simulink model "ES008A_PwrSply"  (R2013b)
settings: Solver=FixedStepDiscrete  SolverMode=SingleTasking  StartTime=0.0  StopTime=1  FixedStep=0.002  RelTol=1e-3
values from neighbouring files (symbols this model uses):
  DiagcReg0Err = DataDict.NTC    [ES008A_PwrSply_DataDict.m]
  DiagcReg1Err = DataDict.NTC    [ES008A_PwrSply_DataDict.m]
  PWRSPLYDIAGREG0READVAL_CNT_U16 = DataDict.Constant    [ES008A_PwrSply_DataDict.m]
  PWRSPLYDIAGREG1READVAL_CNT_U16 = DataDict.Constant    [ES008A_PwrSply_DataDict.m]
  PwrSplyNtc0x07BFailStep = DataDict.Calibration    [ES008A_PwrSply_DataDict.m]
  PwrSplyNtc0x07BPassStep = DataDict.Calibration    [ES008A_PwrSply_DataDict.m]
  PwrSplyNtc0x07CFailStep = DataDict.Calibration    [ES008A_PwrSply_DataDict.m]
  PwrSplyNtc0x07CPassStep = DataDict.Calibration    [ES008A_PwrSply_DataDict.m]
  PwrSplyNtc0x07DFailStep = DataDict.Calibration    [ES008A_PwrSply_DataDict.m]
  PwrSplyNtc0x07DPassStep = DataDict.Calibration    [ES008A_PwrSply_DataDict.m]
  PWRSPLYOUTPENAWRVAL_CNT_U16 = DataDict.Constant    [ES008A_PwrSply_DataDict.m]
  PWRSPLYVRFYRESREG0READVAL_CNT_U16 = DataDict.Constant    [ES008A_PwrSply_DataDict.m]
  PWRSPLYVRFYRESREG1READVAL_CNT_U16 = DataDict.Constant    [ES008A_PwrSply_DataDict.m]
  SerlErr = DataDict.NTC    [ES008A_PwrSply_DataDict.m]
  SpiConf_SpiChannel_PwrSplyCh1 = DataDict.Constant    [ES008A_PwrSply_DataDict.m]
  SpiConf_SpiChannel_PwrSplyCh2 = DataDict.Constant    [ES008A_PwrSply_DataDict.m]
  SpiConf_SpiChannel_PwrSplyCh3 = DataDict.Constant    [ES008A_PwrSply_DataDict.m]
  SpiConf_SpiChannel_PwrSplyCh4 = DataDict.Constant    [ES008A_PwrSply_DataDict.m]
  SpiConf_SpiChannel_PwrSplyCh5 = DataDict.Constant    [ES008A_PwrSply_DataDict.m]
  SpiConf_SpiSequence_PwrSplySeq1 = DataDict.Constant    [ES008A_PwrSply_DataDict.m]
  SpiConf_SpiSequence_PwrSplySeq2 = DataDict.Constant    [ES008A_PwrSply_DataDict.m]
  SpiConf_SpiSequence_PwrSplySeq3 = DataDict.Constant    [ES008A_PwrSply_DataDict.m]
  SpiConf_SpiSequence_PwrSplySeq4 = DataDict.Constant    [ES008A_PwrSply_DataDict.m]
  SpiConf_SpiSequence_PwrSplySeq5 = DataDict.Constant    [ES008A_PwrSply_DataDict.m]
  StrtUpSelfTestReg0Err = DataDict.NTC    [ES008A_PwrSply_DataDict.m]
  StrtUpSelfTestReg1Err = DataDict.NTC    [ES008A_PwrSply_DataDict.m]
undefined symbols (not defined in the file or in its folder): sigbuilder_block, SysSt1
libraries: simulink x11
(part 1 of 4)
settings Model: Creator=HZY4G9  LastModifiedBy=fz41t8
settings SolverCC: AutoInsertRateTranBlk=on  InsertRTBMode=Always
settings DataIOCC: LimitDataPoints=off  SaveFormat=Structure  ReturnWorkspaceOutputs=on
settings OptimizationCC: BlockReduction=off  InlineParams=on  ZeroExternalMemoryAtStartup=off  ZeroInternalMemoryAtStartup=off  OptimizeModelRefInitCode=on  LifeSpan=1
settings DebuggingCC: SignalInfNanChecking=error  SignalRangeChecking=warning  UnderspecifiedInitializationDetection=Simplified  SolverPrmCheckMsg=error  InheritedTsInSrcMsg=error  DiscreteInheritContinuousMsg=error  SingleTaskRateTransMsg=error  TasksWithSamePriorityMsg=error  SigSpecEnsureSampleTimeMsg=error  CheckMatrixSingularityMsg=error  ParameterUnderflowMsg=error  ParameterPrecisionLossMsg=error  ParameterTunabilityLossMsg=error  FixptConstUnderflowMsg=warning  FixptConstOverflowMsg=warning  VectorMatrixConversionMsg=error  SignalLabelMismatchMsg=error  UnconnectedInputMsg=error  UnconnectedOutputMsg=error  UnconnectedLineMsg=error  SFcnCompatibilityMsg=error  UniqueDataStoreMsg=warning  BusObjectLabelMismatch=error  RootOutportRequireBusObject=error  AssertControl=DisableAll  ModelReferenceIOMsg=error  ModelReferenceVersionMismatchMessage=warning  ModelReferenceIOMismatchMessage=error  ModelReferenceCSMismatchMessage=warning  ModelReferenceDataLoggingMessage=error  StateNameClashWarn=warning  StrictBusMsg=ErrorOnBusTreatedAsVector  NonBusSignalsTreatedAsBus=error  SFUnexpectedBacktrackingDiag=error  SFInvalidInputDataAccessInChartInitDiag=error  SFNoUnconditionalDefaultTransitionDiag=error  SFTransitionOutsideNaturalParentDiag=error  SFUnconditionalTransitionShadowingDiag=error  SFUndirectedBroadcastEventsDiag=error
settings ModelReferenceCC: ModelReferenceNumInstancesAllowed=Single
settings RTWCC: SystemTargetFile=autosar.tlc  GenCodeOnly=on  TemplateMakefile=ert_default_tmf  Description=AUTOSAR  GenerateReport=on  ProcessScript=autosar_make_rtw_hook  LaunchReport=on
settings CodeAppCC: GenerateComments=off  IgnoreCustomStorageClasses=off  CustomSymbolStrType=$N$R$M  CustomSymbolStrBlkIO=$N$M  SimulinkBlockComments=off
settings STFCustomTargetCC: ParMdlRefBuildCompliant=on  CompOptLevelCompliant=on  IncludeMdlTerminateFcn=off  CombineOutputUpdateFcns=on  SuppressErrorStatus=on  ERTFirstTimeCompliant=on  ERTCustomFileBanners=on  SupportNonFinite=off  SupportComplex=off  SupportContinuousTime=off  SupportNonInlinedSFcns=off  MATLABClassNameForMDSCustomization=Simulink.SoftwareTarget.ERTCustomization  AutosarCompliant=on  GRTInterface=off  SystemTargetFile=autosar.tlc
settings ERTTargetCC: CodeReplacementLibrary=ANSI_C  ConcurrentExecutionCompliant=off  IncludeMdlTerminateFcn=off  SuppressErrorStatus=on  SupportNonFinite=off  SupportComplex=off  ModelStepFunctionPrototypeControlCompliant=off  CPPClassGenCompliant=off  AutosarCompliant=on  InlinedParameterPlacement=NonHierarchical  ERTCustomFileTemplate=example_file_process.tlc  EnableUserReplacementTypes=on

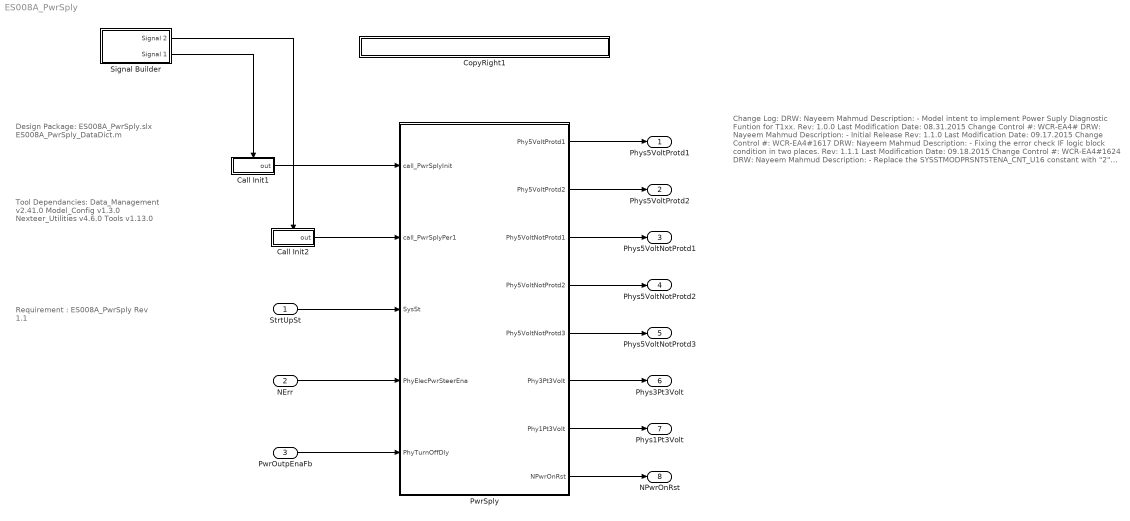
== system ES008A_PwrSply ==
  note: Design Package:
      |
      | ES008A_PwrSply.slx
      | ES008A_PwrSply_DataDict.m
  note: Tool Dependancies:
      |
      | Data_Management v2.41.0
      | Model_Config v1.3.0
      | Nexteer_Utilities v4.6.0
      | Tools v1.13.0
  note: Requirement :
      | ES008A_PwrSply Rev 1.1
  note: Change Log:
      |
      | DRW: Nayeem Mahmud
      | Description:
      | - Model intent to implement Power Suply Diagnostic Funtion for T1xx.
      |
      | Rev: 1.0.0
      | Last Modification Date: 08.31.2015
      | Change Control #: WCR-EA4#
      | DRW: Nayeem Mahmud
      | Description:
      | - Initial Release
      |
      | Rev: 1.1.0
      | Last Modification Date: 09.17.2015
      | Change Control #: WCR-EA4#1617
      | DRW: Nayeem Mahmud
      | Description:
      | - Fixing the error check IF logic block condition in two places.
      |
      | Rev: 1.1.1
      | Last Modification Date: 09.18.2015
      | Change Control #: WCR-EA4#1624
      | DRW: Nayeem Mahmud
      | Description:
      | - Replace the SYSSTMODPRSNTSTENA_CNT_U16 constant with "2"
      |
      |
      | Rev: 1.2.0
      | Last Modification Date: 10.15.2015
      | Change Control #: Anomaly # EA4#1935, Component # 1909, 	WCR-EA4#2035
      | DRW: Nayeem Mahmud
      | Description:
      | - Logic to check both the Diag Reg 0 and Diag Reg 1 has been chaged.
      | - Bit masking value to check the Diag Reg 0 error has been corrected.
      |
      |
      | Rev: 1.3.0
      | Last Modification Date: 03.28.2016
      | Change Control #: CR # EA4#4053, Component # 4875, 	WCR-EA4#4978
      | DRW: Nayeem Mahmud
      | Description:
      | - Adding the functionality to report out the results of start up self test
      | - Two new NTCs 0x07E and 0x07F have been added for this.
      |
      | Rev: 1.4.0
      | Last Modification Date: 04.01.2016
      | Change Control #: CR # EA4#4053, Component # 4875, 	WCR-EA4#5090
      | DRW: Nayeem Mahmud
      | Description:
      | - Fixed the issue with the NtcStsInfo (added a NOT block) in two places
      |
      | Rev: 1.5.0
      | Last Modification Date: 09.09.2016
      | Change Control #: Anomaly # EA4#7193, Component # 7351, 	WCR-EA4#7357
      | DRW: Raghavendran Mohan
      | Description: DataDict.m file change
      | - In DataDict.m file, Changed NTC_0x07D type from 'None' to 'Deb'.
      | - Datatype mismatch fixed in model.
  StrtUpSt : Inport
  NErr : Inport  RequirementInfo={} %GIDa_2993b951_5bd9_4343_99c5_19d61f2e9c43  Port=2
  PwrOutpEnaFb : Inport  RequirementInfo={} %GIDa_e3163a5b_cd98_472f_996c_9901694aa30f  Port=3
  Call Init1 : Subsystem  TreatAsAtomicUnit=on
  Call Init2 : Subsystem  TreatAsAtomicUnit=on
  CopyRight1 : Subsystem  Description=|  mask(Copyright Information){none=on}
      | Copyright info block.                                               
      |                                                                     
      | Place copyright information at the top of every subsystem in design.
      mask prompts: none "No parameters"
      mask help: Place copyright information at the top of every subsystem in design.
      mask Display:
      | NxtrConf = 'Nexteer Confidential';
      | 
      | sys = bdroot; %handle for the current model ("system")
      | first = get_param(sys,'Created');
      | first = first(end-3:end);  %year is last four digits
      | 
      | last = get_param(sys,'LastModifiedDate');
      | if isempty(last)
      |     last = datestr(now,'yyyy');
      | else
      |     last = last(end-3:end);
      | end
      | 
      | if strcmp(first,last)
      |     fprintf('%s -- Copyright %s Nexteer',NxtrConf,first)
      | else
      |     fprintf('%s -- %s%s- %s Nexteer',NxtrConf,char(169),first,last)
      | end
  PwrSply : Subsystem  RequirementInfo={'linktype_rmi_doors' '0000cf50 (/ESG Group/FDD Module Requirements/EA4 Specific/ES008A - PwrSply)' '#ES008A_9' 'true' 'REQ: ES008A_9' '' } %GIDa_d95d113b_b32a_49cc_8d78_f5fb2b103391
  Signal Builder : Subsystem  Tag=STV Subsys  LoadFcn=sigbuilder_block('load');  StartFcn=sigbuilder_block('start');  StopFcn=sigbuilder_block('stop');  ClipboardFcn=sigbuilder_block('clipboard');  mask(Sigbuilder block){}
      mask help: Simulink:masks:SigbuilderBlock_MD
      mask init:
      | if ~strcmp(get_param(bdroot(gcbh),'SimulationStatus'),'stopped') tuvar = sigbuilder_block('maskInit'); end
      settings: CopyFcn=sigbuilder_block('copy');  DeleteFcn=sigbuilder_block('delete');  ModelCloseFcn=sigbuilder_block('modelClose');  PreSaveFcn=sigbuilder_block('preSave');  PauseFcn=sigbuilder_block('pause');  ContinueFcn=sigbuilder_block('continue');  NameChangeFcn=sigbuilder_block('namechange');  OpenFcn=sigbuilder_block('open',[437.25 118.5 550.5 394.5 ]);  CloseFcn=sigbuilder_block('close');
      mask Display: plot(0, 0, 100, 100,[2, 2, 32, 32, 2], [68, 8, 8, 68, 68],[32, 2], [38, 38], [32, 19, 2],[53, 60, 44], [32, 17, 17, 2],[16, 16, 31, 31]);txt = getActiveGroup(gcbh);text(2, 100, txt,'verticalAlignment', 'top');
  Phys5VoltProtd1 : Outport  RequirementInfo={} %GIDa_9f9197d1_ed5a_4c41_8a76_de9d6fef9792
  Phys5VoltProtd2 : Outport  RequirementInfo={} %GIDa_938d4fd1_3ac3_4793_b912_afdca794ca4f  Port=2
  Phys5VoltNotProtd1 : Outport  RequirementInfo={} %GIDa_228821f1_bd9a_4240_92e9_ff558baf1d0e  Port=3
  Phys5VoltNotProtd2 : Outport  RequirementInfo={} %GIDa_8fb49e04_bd98_4471_8ea0_c4f5327ddfa7  Port=4
  Phys5VoltNotProtd3 : Outport  RequirementInfo={} %GIDa_af18e42d_2419_43ef_b731_5edbbe9cdf44  Port=5
  Phys3Pt3Volt : Outport  RequirementInfo={} %GIDa_48afd210_6565_48c9_a60b_4ceb75d4e062  Port=6
  Phys1Pt3Volt : Outport  RequirementInfo={} %GIDa_eb4dff9a_a239_4f61_a51e_94ba26e9c3fe  Port=7
  NPwrOnRst : Outport  RequirementInfo={} %GIDa_906daaee_44a5_4a55_9c03_098358a5c2d2  Port=8
  wires:
  NErr/1 -> PwrSply/4(PhyElecPwrSteerEna)
  PwrOutpEnaFb/1 -> PwrSply/5(PhyTurnOffDly)
  PwrSply/1(Phy5VoltProtd1) -> Phys5VoltProtd1/1
  PwrSply/2(Phy5VoltProtd2) -> Phys5VoltProtd2/1
  PwrSply/3(Phy5VoltNotProtd1) -> Phys5VoltNotProtd1/1
  PwrSply/4(Phy5VoltNotProtd2) -> Phys5VoltNotProtd2/1
  PwrSply/5(Phy5VoltNotProtd3) -> Phys5VoltNotProtd3/1
  PwrSply/6(Phy3Pt3Volt) -> Phys3Pt3Volt/1
  PwrSply/7(Phy1Pt3Volt) -> Phys1Pt3Volt/1
  PwrSply/8(NPwrOnRst) -> NPwrOnRst/1
  Call Init1/1(out) -> PwrSply/1(call_PwrSplyInit)
  StrtUpSt/1 -> PwrSply/3(SysSt)
  Signal Builder/2(Signal 1) -> Call Init1/Enable
  Call Init2/1(out) -> PwrSply/2(call_PwrSplyPer1)
  Signal Builder/1(Signal 2) -> Call Init2/Enable

== system ES008A_PwrSply/Call Init1 ==
  Enable : EnablePort
  Function Call Trigger : simulink/Ports & Subsystems/Function-Call Generator  RequirementInfo={} %GIDa_ff755a2e_49d1_45f7_8591_3ce0ef475338  sample_time=0.002  numberOfIterations=1
  out : Outport
  wires:
  Function Call Trigger/1 -> out/1

== system ES008A_PwrSply/Call Init2 ==
  Enable : EnablePort
  Function Call Trigger : simulink/Ports & Subsystems/Function-Call Generator  RequirementInfo={} %GIDa_6dd05ab1_f91b_4d7a_a0ec_1170d213fa7b  sample_time=0.004  numberOfIterations=1
  out : Outport
  wires:
  Function Call Trigger/1 -> out/1

== system ES008A_PwrSply/CopyRight1 ==

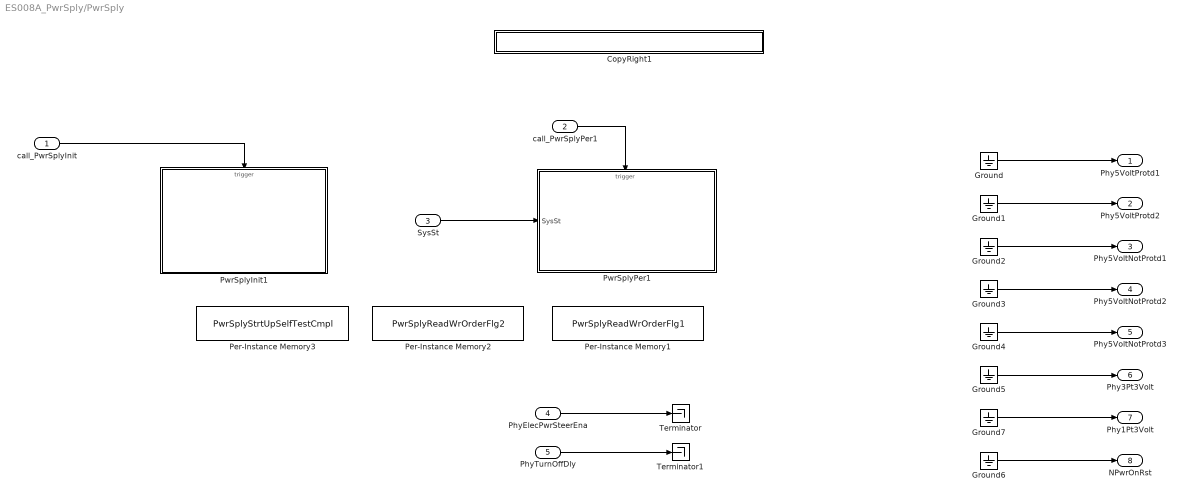
== system ES008A_PwrSply/PwrSply ==
  call_PwrSplyInit : Inport
  call_PwrSplyPer1 : Inport  Port=2
  SysSt : Inport  RequirementInfo={'linktype_rmi_doors' '0000cf50 (/ESG Group/FDD Module Requirements/EA4 Specific/ES008A - PwrSply)' '#ES008A_18' 'true' 'REQ: ES008A_18' '' } %GIDa_c29d43ec_8437_4b86_8b9f_d60d9d0f8c1f  Port=3
  PhyElecPwrSteerEna : Inport  RequirementInfo={'linktype_rmi_doors' '0000cf50 (/ESG Group/FDD Module Requirements/EA4 Specific/ES008A - PwrSply)' '#ES008A_48' 'true' 'REQ: ES008A_48' '' } %GIDa_79fa6cba_2b73_4419_8685_4b91107c24b4  Port=4
  PhyTurnOffDly : Inport  RequirementInfo={'linktype_rmi_doors' '0000cf50 (/ESG Group/FDD Module Requirements/EA4 Specific/ES008A - PwrSply)' '#ES008A_49' 'true' 'REQ: ES008A_49' '' } %GIDa_885462f6_e37b_4022_a155_e2678b5eb9fc  Port=5
  CopyRight1 : Subsystem  Description=|  mask(Copyright Information){none=on}
      | Copyright info block.                                               
      |                                                                     
      | Place copyright information at the top of every subsystem in design.
      mask prompts: none "No parameters"
      mask help: Place copyright information at the top of every subsystem in design.
      mask Display:
      | NxtrConf = 'Nexteer Confidential';
      | 
      | sys = bdroot; %handle for the current model ("system")
      | first = get_param(sys,'Created');
      | first = first(end-3:end);  %year is last four digits
      | 
      | last = get_param(sys,'LastModifiedDate');
      | if isempty(last)
      |     last = datestr(now,'yyyy');
      | else
      |     last = last(end-3:end);
      | end
      | 
      | if strcmp(first,last)
      |     fprintf('%s -- Copyright %s Nexteer',NxtrConf,first)
      | else
      |     fprintf('%s -- %s%s- %s Nexteer',NxtrConf,char(169),first,last)
      | end
  Ground{,1..7} (8 alike) : Ground
  Per-Instance Memory1 : DataStoreMemory  DataStoreName=PwrSplyReadWrOrderFlg1  StateMustResolveToSignalObject=on
  Per-Instance Memory2 : DataStoreMemory  DataStoreName=PwrSplyReadWrOrderFlg2  StateMustResolveToSignalObject=on
  Per-Instance Memory3 : DataStoreMemory  DataStoreName=PwrSplyStrtUpSelfTestCmpl  StateMustResolveToSignalObject=on
  PwrSplyInit1 : Subsystem
  PwrSplyPer1 : Subsystem  RequirementInfo={'linktype_rmi_doors' '0000cf50 (/ESG Group/FDD Module Requirements/EA4 Specific/ES008A - PwrSply)' '#ES008A_15' 'true' 'REQ: ES008A_15' '' ; 'linktype_rmi_doors' '0000cf50 (/ESG Group/FDD Module Requirements/EA4 Specific/ES008A - PwrSply)' '#ES008A_35' 'true' 'REQ: ES008A_35' '' } %GIDa_21503067_1abd_4975_a083_ff275a15b7aa
  Terminator : Terminator
  Terminator1 : Terminator
  Phy5VoltProtd1 : Outport  RequirementInfo={'linktype_rmi_doors' '0000cf50 (/ESG Group/FDD Module Requirements/EA4 Specific/ES008A - PwrSply)' '#ES008A_19' 'true' 'REQ: ES008A_19' '' } %GIDa_2fa7649d_b358_4c36_86cb_a2a2cc9363e6
  Phy5VoltProtd2 : Outport  RequirementInfo={'linktype_rmi_doors' '0000cf50 (/ESG Group/FDD Module Requirements/EA4 Specific/ES008A - PwrSply)' '#ES008A_51' 'true' 'REQ: ES008A_51' '' } %GIDa_a84582b9_42eb_4055_b328_d623692744db  Port=2
  Phy5VoltNotProtd1 : Outport  RequirementInfo={'linktype_rmi_doors' '0000cf50 (/ESG Group/FDD Module Requirements/EA4 Specific/ES008A - PwrSply)' '#ES008A_52' 'true' 'REQ: ES008A_52' '' } %GIDa_452b6491_11ce_4c30_af1c_e28e0f5217d6  Port=3
  Phy5VoltNotProtd2 : Outport  RequirementInfo={'linktype_rmi_doors' '0000cf50 (/ESG Group/FDD Module Requirements/EA4 Specific/ES008A - PwrSply)' '#ES008A_68' 'true' 'REQ: ES008A_68' '' } %GIDa_9ee164d8_2a31_46c2_8fd2_111ec070654d  Port=4
  Phy5VoltNotProtd3 : Outport  RequirementInfo={'linktype_rmi_doors' '0000cf50 (/ESG Group/FDD Module Requirements/EA4 Specific/ES008A - PwrSply)' '#ES008A_67' 'true' 'REQ: ES008A_67' '' } %GIDa_c97b8bc3_d281_460d_8330_8a979dcea7d4  Port=5
  Phy3Pt3Volt : Outport  RequirementInfo={'linktype_rmi_doors' '0000cf50 (/ESG Group/FDD Module Requirements/EA4 Specific/ES008A - PwrSply)' '#ES008A_66' 'true' 'REQ: ES008A_66' '' } %GIDa_fd728fb8_c0bb_4d4c_a9c5_090cba2068e0  Port=6
  Phy1Pt3Volt : Outport  RequirementInfo={'linktype_rmi_doors' '0000cf50 (/ESG Group/FDD Module Requirements/EA4 Specific/ES008A - PwrSply)' '#ES008A_65' 'true' 'REQ: ES008A_65' '' } %GIDa_4da824d7_74ac_4436_8dd2_da7e94321021  Port=7
  NPwrOnRst : Outport  RequirementInfo={'linktype_rmi_doors' '0000cf50 (/ESG Group/FDD Module Requirements/EA4 Specific/ES008A - PwrSply)' '#ES008A_69' 'true' 'REQ: ES008A_69' '' } %GIDa_42175ed4_51f9_467f_9b8d_a07c48cc90f3  Port=8
  wires:
  call_PwrSplyPer1/1 -> PwrSplyPer1/Trigger
  Ground/1 -> Phy5VoltProtd1/1
  SysSt/1 -> PwrSplyPer1/1(SysSt)
  PhyElecPwrSteerEna/1 -> Terminator/1
  PhyTurnOffDly/1 -> Terminator1/1
  Ground1/1 -> Phy5VoltProtd2/1
  Ground2/1 -> Phy5VoltNotProtd1/1
  Ground3/1 -> Phy5VoltNotProtd2/1
  Ground4/1 -> Phy5VoltNotProtd3/1
  Ground5/1 -> Phy3Pt3Volt/1
  Ground6/1 -> NPwrOnRst/1
  Ground7/1 -> Phy1Pt3Volt/1
  call_PwrSplyInit/1 -> PwrSplyInit1/Trigger

== system ES008A_PwrSply/Signal Builder ==
  Demux : Demux  Tag=STV Demux  Outputs=2
  FromWs : FromWorkspace  Tag=STV FromWs  VariableName=tuvar  SampleTime=0
      SigBuilderData=|
      | common.afterFinalStr = 'Extrapolate'
      | common.sampleTime = 0
      | dataSet.timeRange = [0 1]
      | dataSet.name = 'Group 1'
      | sbobj.Groups.Name = 'Group 1'
      | sbobj.Groups.Signals(1).Name = 'Signal 2'
      | sbobj.Groups.Signals(1).XData = [0 0.02 0.02 1]
      | sbobj.Groups.Signals(1).YData = [0 0 1 1]
      | sbobj.Groups.Signals(2).Name = 'Signal 1'
      | sbobj.Groups.Signals(2).XData = [0 0.01 0.01 1]
      | sbobj.Groups.Signals(2).YData = [1 1 0 0]
      | sbobj.Groups.TimeRange = [0 1]
  Signal 2 : Outport  Tag=STV Outport
  Signal 1 : Outport  Tag=STV Outport  Port=2
  wires:
  FromWs/1 -> Demux/1
  Demux/1 -> Signal 2/1
  Demux/2 -> Signal 1/1

== system ES008A_PwrSply/PwrSply/CopyRight1 ==

== system ES008A_PwrSply/PwrSply/PwrSplyInit1 ==
  function : TriggerPort  TriggerType=function-call
  Constant1 : Constant  Value=0  OutDataTypeStr=boolean
  Constant2 : Constant  Value=0  OutDataTypeStr=boolean
  Constant3 : Constant  Value=0  OutDataTypeStr=boolean
  CopyRight1 : Subsystem  Description=|  mask(Copyright Information){none=on}
      | Copyright info block.                                               
      |                                                                     
      | Place copyright information at the top of every subsystem in design.
      mask prompts: none "No parameters"
      mask help: Place copyright information at the top of every subsystem in design.
      mask Display:
      | NxtrConf = 'Nexteer Confidential';
      | 
      | sys = bdroot; %handle for the current model ("system")
      | first = get_param(sys,'Created');
      | first = first(end-3:end);  %year is last four digits
      | 
      | last = get_param(sys,'LastModifiedDate');
      | if isempty(last)
      |     last = datestr(now,'yyyy');
      | else
      |     last = last(end-3:end);
      | end
      | 
      | if strcmp(first,last)
      |     fprintf('%s -- Copyright %s Nexteer',NxtrConf,first)
      | else
      |     fprintf('%s -- %s%s- %s Nexteer',NxtrConf,char(169),first,last)
      | end
  Data Store Write : DataStoreWrite  DataStoreName=PwrSplyStrtUpSelfTestCmpl
  Data Store Write1 : DataStoreWrite  DataStoreName=PwrSplyReadWrOrderFlg1
  Data Store Write2 : DataStoreWrite  DataStoreName=PwrSplyReadWrOrderFlg2
  wires:
  Constant1/1 -> Data Store Write/1
  Constant2/1 -> Data Store Write1/1
  Constant3/1 -> Data Store Write2/1

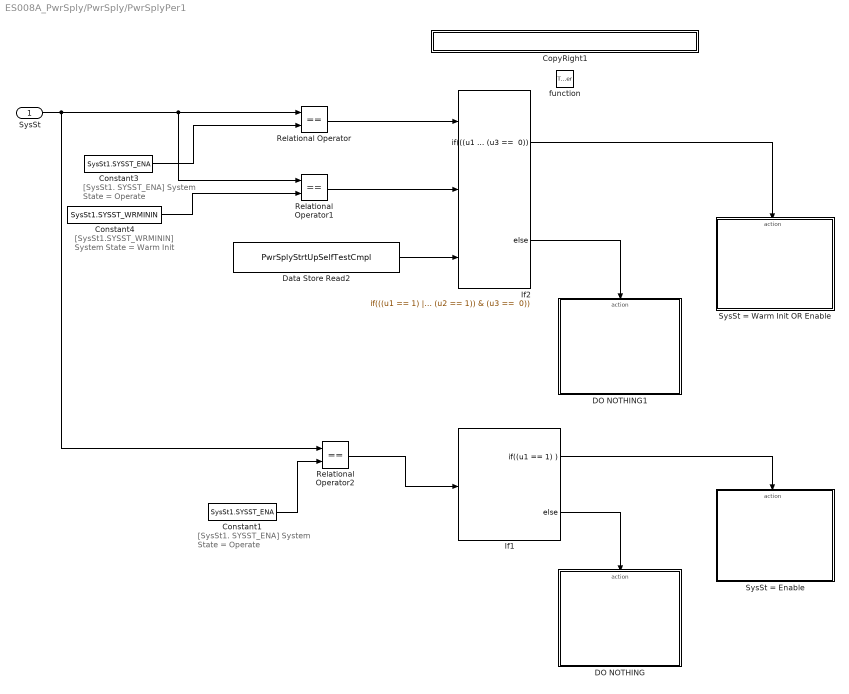
== system ES008A_PwrSply/PwrSply/PwrSplyPer1 ==
  note: [SysSt1. SYSST_ENA]
      | System State = Operate
  note: [SysSt1. SYSST_ENA]
      | System State = Operate
  note: [SysSt1.SYSST_WRMININ]
      |    System State = Warm Init
  SysSt : Inport  RequirementInfo={} %GIDa_5b596eb2_5211_4207_8c2b_8304b28df24a
  function : TriggerPort  TriggerType=function-call
  Constant1 : Constant  Value=SysSt1.SYSST_ENA  OutDataTypeStr=Enum: SysSt1
  Constant3 : Constant  Value=SysSt1.SYSST_ENA  OutDataTypeStr=Enum: SysSt1
  Constant4 : Constant  Value=SysSt1.SYSST_WRMININ  OutDataTypeStr=Enum: SysSt1
  CopyRight1 : Subsystem  Description=|  mask(Copyright Information){none=on}
      | Copyright info block.                                               
      |                                                                     
      | Place copyright information at the top of every subsystem in design.
      mask prompts: none "No parameters"
      mask help: Place copyright information at the top of every subsystem in design.
      mask Display:
      | NxtrConf = 'Nexteer Confidential';
      | 
      | sys = bdroot; %handle for the current model ("system")
      | first = get_param(sys,'Created');
      | first = first(end-3:end);  %year is last four digits
      | 
      | last = get_param(sys,'LastModifiedDate');
      | if isempty(last)
      |     last = datestr(now,'yyyy');
      | else
      |     last = last(end-3:end);
      | end
      | 
      | if strcmp(first,last)
      |     fprintf('%s -- Copyright %s Nexteer',NxtrConf,first)
      | else
      |     fprintf('%s -- %s%s- %s Nexteer',NxtrConf,char(169),first,last)
      | end
  DO NOTHING : Subsystem
  DO NOTHING1 : Subsystem
  Data Store Read2 : DataStoreRead  DataStoreName=PwrSplyStrtUpSelfTestCmpl
  If1 : If  RequirementInfo={'linktype_rmi_doors' '0000cf50 (/ESG Group/FDD Module Requirements/EA4 Specific/ES008A - PwrSply)' '#ES008A_70' 'true' 'REQ: ES008A_70' '' } %GIDa_e4499870_91b3_40c8_a94a_0d57718268f0  IfExpression=(u1 == 1)
  If2 : If  RequirementInfo={} %GIDa_7280bc1c_0da5_4fb0_b0e3_5c99ce7504d9  NumInputs=3  IfExpression="((u1 == 1) | (u2 == 1)) & (u3 ==  0)"
  Relational Operator : RelationalOperator  Operator===  OutDataTypeStr=boolean
  Relational Operator1 : RelationalOperator  Operator===  OutDataTypeStr=boolean
  Relational Operator2 : RelationalOperator  Operator===  OutDataTypeStr=boolean
  SysSt = Enable : Subsystem  RequirementInfo={'linktype_rmi_doors' '0000cf50 (/ESG Group/FDD Module Requirements/EA4 Specific/ES008A - PwrSply)' '#ES008A_70' 'true' 'REQ: ES008A_70' '' } %GIDa_f09ed0ff_e7dd_4660_a710_5e7ade943f34
  SysSt = Warm Init OR Enable : Subsystem  RequirementInfo={} %GIDa_9cb12e74_1a07_4738_ab06_ee8fb2c18ce7
  wires:
  If1/1 -> SysSt = Enable/Action
  If1/2 -> DO NOTHING/Action
  SysSt/1 -> Relational Operator2/1, Relational Operator1/1, Relational Operator/1
  If2/1 -> SysSt = Warm Init OR Enable/Action
  If2/2 -> DO NOTHING1/Action
  Data Store Read2/1 -> If2/3
  Constant3/1 -> Relational Operator/2
  Relational Operator/1 -> If2/1
  Constant4/1 -> Relational Operator1/2
  Relational Operator1/1 -> If2/2
  Relational Operator2/1 -> If1/1
  Constant1/1 -> Relational Operator2/2

== system ES008A_PwrSply/PwrSply/PwrSplyInit1/CopyRight1 ==

== system ES008A_PwrSply/PwrSply/PwrSplyPer1/CopyRight1 ==

== system ES008A_PwrSply/PwrSply/PwrSplyPer1/DO NOTHING ==
  note: Do Nothing
  Action Port : ActionPort  ActionType=else
  CopyRight1 : Subsystem  Description=|  mask(Copyright Information){none=on}
      | Copyright info block.                                               
      |                                                                     
      | Place copyright information at the top of every subsystem in design.
      mask prompts: none "No parameters"
      mask help: Place copyright information at the top of every subsystem in design.
      mask Display:
      | NxtrConf = 'Nexteer Confidential';
      | 
      | sys = bdroot; %handle for the current model ("system")
      | first = get_param(sys,'Created');
      | first = first(end-3:end);  %year is last four digits
      | 
      | last = get_param(sys,'LastModifiedDate');
      | if isempty(last)
      |     last = datestr(now,'yyyy');
      | else
      |     last = last(end-3:end);
      | end
      | 
      | if strcmp(first,last)
      |     fprintf('%s -- Copyright %s Nexteer',NxtrConf,first)
      | else
      |     fprintf('%s -- %s%s- %s Nexteer',NxtrConf,char(169),first,last)
      | end

== system ES008A_PwrSply/PwrSply/PwrSplyPer1/DO NOTHING1 ==
  note: Do Nothing
  Action Port : ActionPort  ActionType=else
  CopyRight1 : Subsystem  Description=|  mask(Copyright Information){none=on}
      | Copyright info block.                                               
      |                                                                     
      | Place copyright information at the top of every subsystem in design.
      mask prompts: none "No parameters"
      mask help: Place copyright information at the top of every subsystem in design.
      mask Display:
      | NxtrConf = 'Nexteer Confidential';
      | 
      | sys = bdroot; %handle for the current model ("system")
      | first = get_param(sys,'Created');
      | first = first(end-3:end);  %year is last four digits
      | 
      | last = get_param(sys,'LastModifiedDate');
      | if isempty(last)
      |     last = datestr(now,'yyyy');
      | else
      |     last = last(end-3:end);
      | end
      | 
      | if strcmp(first,last)
      |     fprintf('%s -- Copyright %s Nexteer',NxtrConf,first)
      | else
      |     fprintf('%s -- %s%s- %s Nexteer',NxtrConf,char(169),first,last)
      | end

== system ES008A_PwrSply/PwrSply/PwrSplyPer1/SysSt = Enable ==
  Action Port : ActionPort  ActionType=then
  CopyRight1 : Subsystem  Description=|  mask(Copyright Information){none=on}
      | Copyright info block.                                               
      |                                                                     
      | Place copyright information at the top of every subsystem in design.
      mask prompts: none "No parameters"
      mask help: Place copyright information at the top of every subsystem in design.
      mask Display:
      | NxtrConf = 'Nexteer Confidential';
      | 
      | sys = bdroot; %handle for the current model ("system")
      | first = get_param(sys,'Created');
      | first = first(end-3:end);  %year is last four digits
      | 
      | last = get_param(sys,'LastModifiedDate');
      | if isempty(last)
      |     last = datestr(now,'yyyy');
      | else
      |     last = last(end-3:end);
      | end
      | 
      | if strcmp(first,last)
      |     fprintf('%s -- Copyright %s Nexteer',NxtrConf,first)
      | else
      |     fprintf('%s -- %s%s- %s Nexteer',NxtrConf,char(169),first,last)
      | end
  Data Store Read1 : DataStoreRead  DataStoreName=PwrSplyReadWrOrderFlg1
  If1 : If  IfExpression=u1 == 0
  "PwrSplyReadWrOrderFlg1 = 0 (Write Cmd to get Diag Status) " : Subsystem  RequirementInfo={'linktype_rmi_doors' '0000cf50 (/ESG Group/FDD Module Requirements/EA4 Specific/ES008A_PwrSply)' '#ES008A_109' 'true' 'REQ: ES008A_109' '' } %GIDa_9c80e880_f77f_439c_9df0_b85375d3c3f6
  PwrSplyReadWrOrderFlg1 = 1 (Read Buffer) : Subsystem  RequirementInfo={'linktype_rmi_doors' '0000cf50 (/ESG Group/FDD Module Requirements/EA4 Specific/ES008A_PwrSply)' '#ES008A_111' 'true' 'REQ: ES008A_111' '' } %GIDa_2594ab7f_e454_446f_9943_d559df18bdb1
  wires:
  If1/1 -> "PwrSplyReadWrOrderFlg1 = 0 (Write Cmd to get Diag Status) "/Action
  If1/2 -> PwrSplyReadWrOrderFlg1 = 1 (Read Buffer)/Action
  Data Store Read1/1 -> If1/1

== system ES008A_PwrSply/PwrSply/PwrSplyPer1/SysSt = Warm Init OR Enable ==
  Action Port : ActionPort  ActionType=then
  CopyRight1 : Subsystem  Description=|  mask(Copyright Information){none=on}
      | Copyright info block.                                               
      |                                                                     
      | Place copyright information at the top of every subsystem in design.
      mask prompts: none "No parameters"
      mask help: Place copyright information at the top of every subsystem in design.
      mask Display:
      | NxtrConf = 'Nexteer Confidential';
      | 
      | sys = bdroot; %handle for the current model ("system")
      | first = get_param(sys,'Created');
      | first = first(end-3:end);  %year is last four digits
      | 
      | last = get_param(sys,'LastModifiedDate');
      | if isempty(last)
      |     last = datestr(now,'yyyy');
      | else
      |     last = last(end-3:end);
      | end
      | 
      | if strcmp(first,last)
      |     fprintf('%s -- Copyright %s Nexteer',NxtrConf,first)
      | else
      |     fprintf('%s -- %s%s- %s Nexteer',NxtrConf,char(169),first,last)
      | end
  Data Store Read1 : DataStoreRead  DataStoreName=PwrSplyReadWrOrderFlg2
  If1 : If  IfExpression=u1 == 0
  "PwrSplyReadWrOrderFlg2 = 0 (Write Cmd to get Diag Status) " : Subsystem  RequirementInfo={'linktype_rmi_doors' '0000cf50 (/ESG Group/FDD Module Requirements/EA4 Specific/ES008A_PwrSply)' '#ES008A_107' 'true' 'REQ: ES008A_107' '' } %GIDa_ea804c10_9799_4e6e_b30b_b693c4b35637
  PwrSplyReadWrOrderFlg2 = 1 (Read Buffer) : Subsystem  RequirementInfo={'linktype_rmi_doors' '0000cf50 (/ESG Group/FDD Module Requirements/EA4 Specific/ES008A_PwrSply)' '#ES008A_108' 'true' 'REQ: ES008A_108' '' } %GIDa_087b366a_2c10_46c6_b56c_1610462d32ed
  wires:
  Data Store Read1/1 -> If1/1
  If1/2 -> PwrSplyReadWrOrderFlg2 = 1 (Read Buffer)/Action
  If1/1 -> "PwrSplyReadWrOrderFlg2 = 0 (Write Cmd to get Diag Status) "/Action

== system ES008A_PwrSply/PwrSply/PwrSplyPer1/DO NOTHING/CopyRight1 ==

== system ES008A_PwrSply/PwrSply/PwrSplyPer1/DO NOTHING1/CopyRight1 ==

== system ES008A_PwrSply/PwrSply/PwrSplyPer1/SysSt = Enable/CopyRight1 ==

== system ES008A_PwrSply/PwrSply/PwrSplyPer1/SysSt = Enable/PwrSplyReadWrOrderFlg1 = 0 (Write Cmd to get Diag Status)  ==
  note: Implement in this order
  note: Channel 1 --> for Write Cmd
      | Channel 2 --> for Diag Register 0
      | Channel 3 --> for Diag Register 1
  Action Port : ActionPort  ActionType=then
  Constant1 : Constant  OutDataTypeStr=boolean
  CopyRight1 : Subsystem  Description=|  mask(Copyright Information){none=on}
      | Copyright info block.                                               
      |                                                                     
      | Place copyright information at the top of every subsystem in design.
      mask prompts: none "No parameters"
      mask help: Place copyright information at the top of every subsystem in design.
      mask Display:
      | NxtrConf = 'Nexteer Confidential';
      | 
      | sys = bdroot; %handle for the current model ("system")
      | first = get_param(sys,'Created');
      | first = first(end-3:end);  %year is last four digits
      | 
      | last = get_param(sys,'LastModifiedDate');
      | if isempty(last)
      |     last = datestr(now,'yyyy');
      | else
      |     last = last(end-3:end);
      | end
      | 
      | if strcmp(first,last)
      |     fprintf('%s -- Copyright %s Nexteer',NxtrConf,first)
      | else
      |     fprintf('%s -- %s%s- %s Nexteer',NxtrConf,char(169),first,last)
      | end
  Data Store Write : DataStoreWrite  DataStoreName=PwrSplyReadWrOrderFlg1
  Read Message 1 : Subsystem  RequirementInfo={'linktype_rmi_doors' '0000cf50 (/ESG Group/FDD Module Requirements/EA4 Specific/ES008A_PwrSply)' '#ES008A_110' 'true' 'REQ: ES008A_110' '' } %GIDa_4e0d9faf_3ebd_40f0_842c_078a8ce0398e
  Read Message 2 : Subsystem  RequirementInfo={'linktype_rmi_doors' '0000cf50 (/ESG Group/FDD Module Requirements/EA4 Specific/ES008A_PwrSply)' '#ES008A_110' 'true' 'REQ: ES008A_110' '' } %GIDa_d49b1de0_36f1_434c_a15e_be2544ef9b57
  Write Message 1 : Subsystem  RequirementInfo={'linktype_rmi_doors' '0000cf50 (/ESG Group/FDD Module Requirements/EA4 Specific/ES008A_PwrSply)' '#ES008A_109' 'true' 'REQ: ES008A_109' '' } %GIDa_a9fe6469_ca1f_4ac7_a9ae_cfb48333e5a0
  wires:
  Constant1/1 -> Data Store Write/1

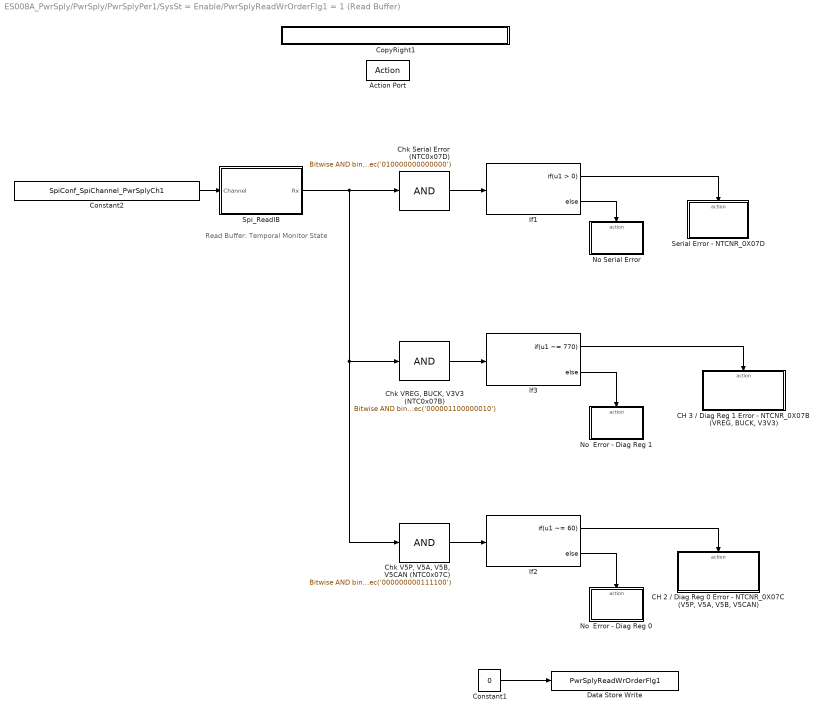
== system ES008A_PwrSply/PwrSply/PwrSplyPer1/SysSt = Enable/PwrSplyReadWrOrderFlg1 = 1 (Read Buffer) ==
  note: Read Buffer: Temporal Monitor State
  Action Port : ActionPort  ActionType=else
  "CH 2 / Diag Reg 0 Error - NTCNR_0X07C (V5P, V5A, V5B, V5CAN)" : Subsystem  RequirementInfo={'linktype_rmi_doors' '0000cf50 (/ESG Group/FDD Module Requirements/EA4 Specific/ES008A - PwrSply)' '#ES008A_91' 'true' 'REQ: ES008A_91' '' ; 'linktype_rmi_doors' '0000cf50 (/ESG Group/FDD Module Requirements/EA4 Specific/ES008A - PwrSply)' '#ES008A_92' 'true' 'REQ: ES008A_92' '' ; 'linktype_rmi_doors' '0000cf50 (/ESG Group/FDD Module Requirements/EA4 Specific/ES008A - PwrSply)' '#ES008A_103' 'true' 'REQ: ES008A_103' '' ; 'linktype_rmi_doors' '0000cf50 (/ESG Group/FDD Module Requirements/EA4 Specific/ES008A - PwrSply)' '#ES008A_104' 'true' 'REQ: ES008A_104' '' ; 'linktype_rmi_doors' '0000cf50 (/ESG Group/FDD Module Requirements/EA4 Specific/ES008A - PwrSply)' '#ES008A_102' 'true' 'REQ: ES008A_102' '' ; 'linktype_rmi_doors' '0000cf50 (/ESG Group/FDD Module Requirements/EA4 Specific/ES008A - PwrSply)' '#ES008A_101' 'true' 'REQ: ES008A_101' '' ; 'linktype_rmi_doors' '0000cf50 (/ESG Group/FDD Module Requirements/EA4 Specific/ES008A - PwrSply)' '#ES008A_100' 'true' 'REQ: ES008A_100' '' ; 'linktype_rmi_doors' '0000cf50 (/ESG Group/FDD Module Requirements/EA4 Specific/ES008A - PwrSply)' '#ES008A_99' 'true' 'REQ: ES008A_99' '' ; 'linktype_rmi_doors' '0000cf50 (/ESG Group/FDD Module Requirements/EA4 Specific/ES008A - PwrSply)' '#ES008A_98' 'true' 'REQ: ES008A_98' '' } %GIDa_aad65a7d_3638_4aa6_b7d8_2de8f64ec733
  "CH 3 / Diag Reg 1 Error - NTCNR_0X07B (VREG, BUCK, V3V3)" : Subsystem  RequirementInfo={'linktype_rmi_doors' '0000cf50 (/ESG Group/FDD Module Requirements/EA4 Specific/ES008A - PwrSply)' '#ES008A_24' 'true' 'REQ: ES008A_24' '' ; 'linktype_rmi_doors' '0000cf50 (/ESG Group/FDD Module Requirements/EA4 Specific/ES008A - PwrSply)' '#ES008A_27' 'true' 'REQ: ES008A_27' '' ; 'linktype_rmi_doors' '0000cf50 (/ESG Group/FDD Module Requirements/EA4 Specific/ES008A - PwrSply)' '#ES008A_28' 'true' 'REQ: ES008A_28' '' ; 'linktype_rmi_doors' '0000cf50 (/ESG Group/FDD Module Requirements/EA4 Specific/ES008A - PwrSply)' '#ES008A_74' 'true' 'REQ: ES008A_74' '' ; 'linktype_rmi_doors' '0000cf50 (/ESG Group/FDD Module Requirements/EA4 Specific/ES008A - PwrSply)' '#ES008A_73' 'true' 'REQ: ES008A_73' '' ; 'linktype_rmi_doors' '0000cf50 (/ESG Group/FDD Module Requirements/EA4 Specific/ES008A - PwrSply)' '#ES008A_72' 'true' 'REQ: ES008A_72' '' ; 'linktype_rmi_doors' '0000cf50 (/ESG Group/FDD Module Requirements/EA4 Specific/ES008A - PwrSply)' '#ES008A_71' 'true' 'REQ: ES008A_71' '' } %GIDa_ac0f842b_0518_4dd3_9fff_b079284210e9
  Chk Serial Error (NTC0x07D) : simulink/Logic and Bit Operations/Bitwise Operator  logicop=AND  UseBitMask=on  BitMask=bin2dec('010000000000000')  BitMaskRealWorld=Stored Integer
  "Chk V5P, V5A, V5B, V5CAN (NTC0x07C)" : simulink/Logic and Bit Operations/Bitwise Operator  logicop=AND  UseBitMask=on  BitMask=bin2dec('000000000111100')  BitMaskRealWorld=Stored Integer
  "Chk VREG, BUCK, V3V3 (NTC0x07B)" : simulink/Logic and Bit Operations/Bitwise Operator  logicop=AND  UseBitMask=on  BitMask=bin2dec('000001100000010')  BitMaskRealWorld=Stored Integer
  Constant1 : Constant  Value=0  OutDataTypeStr=boolean
  Constant2 : Constant  Value=SpiConf_SpiChannel_PwrSplyCh1
  CopyRight1 : Subsystem  Description=|  mask(Copyright Information){none=on}
      | Copyright info block.                                               
      |                                                                     
      | Place copyright information at the top of every subsystem in design.
      mask prompts: none "No parameters"
      mask help: Place copyright information at the top of every subsystem in design.
      mask Display:
      | NxtrConf = 'Nexteer Confidential';
      | 
      | sys = bdroot; %handle for the current model ("system")
      | first = get_param(sys,'Created');
      | first = first(end-3:end);  %year is last four digits
      | 
      | last = get_param(sys,'LastModifiedDate');
      | if isempty(last)
      |     last = datestr(now,'yyyy');
      | else
      |     last = last(end-3:end);
      | end
      | 
      | if strcmp(first,last)
      |     fprintf('%s -- Copyright %s Nexteer',NxtrConf,first)
      | else
      |     fprintf('%s -- %s%s- %s Nexteer',NxtrConf,char(169),first,last)
      | end
  Data Store Write : DataStoreWrite  DataStoreName=PwrSplyReadWrOrderFlg1
  If1 : If
  If2 : If  IfExpression=u1 ~= 60
  If3 : If  IfExpression=u1 ~= 770
  No  Error - Diag Reg 0 : Subsystem  RequirementInfo={'linktype_rmi_doors' '0000cf50 (/ESG Group/FDD Module Requirements/EA4 Specific/ES008A - PwrSply)' '#ES008A_91' 'true' 'REQ: ES008A_91' '' ; 'linktype_rmi_doors' '0000cf50 (/ESG Group/FDD Module Requirements/EA4 Specific/ES008A - PwrSply)' '#ES008A_93' 'true' 'REQ: ES008A_93' '' } %GIDa_b8bb8819_b6ba_4d84_8768_52a4c92c274f
  No  Error - Diag Reg 1 : Subsystem  RequirementInfo={'linktype_rmi_doors' '0000cf50 (/ESG Group/FDD Module Requirements/EA4 Specific/ES008A - PwrSply)' '#ES008A_24' 'true' 'REQ: ES008A_24' '' ; 'linktype_rmi_doors' '0000cf50 (/ESG Group/FDD Module Requirements/EA4 Specific/ES008A - PwrSply)' '#ES008A_30' 'true' 'REQ: ES008A_30' '' } %GIDa_5b056c4c_952f_486b_ac8d_8985a2a38019
  No Serial Error : Subsystem  RequirementInfo={'linktype_rmi_doors' '0000cf50 (/ESG Group/FDD Module Requirements/EA4 Specific/ES008A - PwrSply)' '#ES008A_97' 'true' 'REQ: ES008A_97' '' ; 'linktype_rmi_doors' '0000cf50 (/ESG Group/FDD Module Requirements/EA4 Specific/ES008A - PwrSply)' '#ES008A_94' 'true' 'REQ: ES008A_94' '' } %GIDa_4e8b881b_8c70_4dd5_a92b_65f26be87514
  Serial Error - NTCNR_0X07D : Subsystem  RequirementInfo={'linktype_rmi_doors' '0000cf50 (/ESG Group/FDD Module Requirements/EA4 Specific/ES008A - PwrSply)' '#ES008A_97' 'true' 'REQ: ES008A_97' '' ; 'linktype_rmi_doors' '0000cf50 (/ESG Group/FDD Module Requirements/EA4 Specific/ES008A - PwrSply)' '#ES008A_95' 'true' 'REQ: ES008A_95' '' } %GIDa_ec7c2748_9ee8_4921_9250_ce166c74b7ad
  Spi_ReadIB : Subsystem  RequirementInfo={'linktype_rmi_doors' '0000cf50 (/ESG Group/FDD Module Requirements/EA4 Specific/ES008A_PwrSply)' '#ES008A_109' 'true' 'REQ: ES008A_109' '' } %GIDa_d94459b4_120c_48ef_afed_24db7de4f7c5
  wires:
  Constant1/1 -> Data Store Write/1
  Chk Serial Error (NTC0x07D)/1 -> If1/1
  Spi_ReadIB/1(Rx) -> Chk Serial Error (NTC0x07D)/1, "Chk V5P, V5A, V5B, V5CAN (NTC0x07C)"/1, "Chk VREG, BUCK, V3V3 (NTC0x07B)"/1
  Constant2/1 -> Spi_ReadIB/1(Channel)
  If1/1 -> Serial Error - NTCNR_0X07D/Action
  If1/2 -> No Serial Error/Action
  "Chk VREG, BUCK, V3V3 (NTC0x07B)"/1 -> If3/1
  If3/1 -> "CH 3 / Diag Reg 1 Error - NTCNR_0X07B (VREG, BUCK, V3V3)"/Action
  If3/2 -> No  Error - Diag Reg 1/Action
  "Chk V5P, V5A, V5B, V5CAN (NTC0x07C)"/1 -> If2/1
  If2/1 -> "CH 2 / Diag Reg 0 Error - NTCNR_0X07C (V5P, V5A, V5B, V5CAN)"/Action
  If2/2 -> No  Error - Diag Reg 0/Action

== system ES008A_PwrSply/PwrSply/PwrSplyPer1/SysSt = Warm Init OR Enable/CopyRight1 ==

== system ES008A_PwrSply/PwrSply/PwrSplyPer1/SysSt = Warm Init OR Enable/PwrSplyReadWrOrderFlg2 = 0 (Write Cmd to get Diag Status)  ==
  note: Channel 4 --> for Verify_Result_0 Register
      | Channel 5 --> for Verify_Result_1 Register
  note: Implement in this order
  Action Port : ActionPort  ActionType=then
  Constant1 : Constant  OutDataTypeStr=boolean
  CopyRight1 : Subsystem  Description=|  mask(Copyright Information){none=on}
      | Copyright info block.                                               
      |                                                                     
      | Place copyright information at the top of every subsystem in design.
      mask prompts: none "No parameters"
      mask help: Place copyright information at the top of every subsystem in design.
      mask Display:
      | NxtrConf = 'Nexteer Confidential';
      | 
      | sys = bdroot; %handle for the current model ("system")
      | first = get_param(sys,'Created');
      | first = first(end-3:end);  %year is last four digits
      | 
      | last = get_param(sys,'LastModifiedDate');
      | if isempty(last)
      |     last = datestr(now,'yyyy');
      | else
      |     last = last(end-3:end);
      | end
      | 
      | if strcmp(first,last)
      |     fprintf('%s -- Copyright %s Nexteer',NxtrConf,first)
      | else
      |     fprintf('%s -- %s%s- %s Nexteer',NxtrConf,char(169),first,last)
      | end
  Data Store Write : DataStoreWrite  DataStoreName=PwrSplyReadWrOrderFlg2
  Read Message 1 : Subsystem  RequirementInfo={'linktype_rmi_doors' '0000cf50 (/ESG Group/FDD Module Requirements/EA4 Specific/ES008A_PwrSply)' '#ES008A_107' 'true' 'REQ: ES008A_107' '' } %GIDa_7c658cc9_5d31_4c6d_bff7_5c45aa7b0cb0
  Read Message 2 : Subsystem  RequirementInfo={'linktype_rmi_doors' '0000cf50 (/ESG Group/FDD Module Requirements/EA4 Specific/ES008A_PwrSply)' '#ES008A_107' 'true' 'REQ: ES008A_107' '' } %GIDa_e7aba49e_3e95_42d2_b1d0_2e05932e2c54
  wires:
  Constant1/1 -> Data Store Write/1

== system ES008A_PwrSply/PwrSply/PwrSplyPer1/SysSt = Warm Init OR Enable/PwrSplyReadWrOrderFlg2 = 1 (Read Buffer) ==
  note: Channel 4 --> for Verify_Result_0 Register
      | Channel 5 --> for Verify_Result_1 Register
  Action Port : ActionPort  ActionType=else
  Channel 4 : Subsystem  RequirementInfo={'linktype_rmi_doors' '0000cf50 (/ESG Group/FDD Module Requirements/EA4 Specific/ES008A_PwrSply)' '#ES008A_108' 'true' 'REQ: ES008A_108' '' } %GIDa_8a9e981a_274e_41f8_b8ad_fe148b2ecbb5
  Channel 5 : Subsystem  RequirementInfo={'linktype_rmi_doors' '0000cf50 (/ESG Group/FDD Module Requirements/EA4 Specific/ES008A_PwrSply)' '#ES008A_108' 'true' 'REQ: ES008A_108' '' } %GIDa_b0fc2e3d_e357_4e25_a352_89ecbb375ef4
  Constant1 : Constant  OutDataTypeStr=boolean
  CopyRight1 : Subsystem  Description=|  mask(Copyright Information){none=on}
      | Copyright info block.                                               
      |                                                                     
      | Place copyright information at the top of every subsystem in design.
      mask prompts: none "No parameters"
      mask help: Place copyright information at the top of every subsystem in design.
      mask Display:
      | NxtrConf = 'Nexteer Confidential';
      | 
      | sys = bdroot; %handle for the current model ("system")
      | first = get_param(sys,'Created');
      | first = first(end-3:end);  %year is last four digits
      | 
      | last = get_param(sys,'LastModifiedDate');
      | if isempty(last)
      |     last = datestr(now,'yyyy');
      | else
      |     last = last(end-3:end);
      | end
      | 
      | if strcmp(first,last)
      |     fprintf('%s -- Copyright %s Nexteer',NxtrConf,first)
      | else
      |     fprintf('%s -- %s%s- %s Nexteer',NxtrConf,char(169),first,last)
      | end
  Data Store Write : DataStoreWrite  DataStoreName=PwrSplyStrtUpSelfTestCmpl
  wires:
  Constant1/1 -> Data Store Write/1

== system ES008A_PwrSply/PwrSply/PwrSplyPer1/SysSt = Enable/PwrSplyReadWrOrderFlg1 = 0 (Write Cmd to get Diag Status) /CopyRight1 ==

== system ES008A_PwrSply/PwrSply/PwrSplyPer1/SysSt = Enable/PwrSplyReadWrOrderFlg1 = 0 (Write Cmd to get Diag Status) /Read Message 1 ==
  note: 3072
  note: Channel 1 --> for Write Cmd
      | Channel 2 --> for Diag Register 0
      | Channel 3 --> for Diag Register 1
  note: Read Cmd: Diag Reg 0: 00011 0 0 00000000
  Call_Spi_AsyncTransmit : Subsystem
  Constant2 : Constant  Value=SpiConf_SpiSequence_PwrSplySeq2
  Constant3 : Constant  Value=SpiConf_SpiChannel_PwrSplyCh2
  Constant5 : Constant  Value=PWRSPLYDIAGREG0READVAL_CNT_U16
  CopyRight1 : Subsystem  Description=|  mask(Copyright Information){none=on}
      | Copyright info block.                                               
      |                                                                     
      | Place copyright information at the top of every subsystem in design.
      mask prompts: none "No parameters"
      mask help: Place copyright information at the top of every subsystem in design.
      mask Display:
      | NxtrConf = 'Nexteer Confidential';
      | 
      | sys = bdroot; %handle for the current model ("system")
      | first = get_param(sys,'Created');
      | first = first(end-3:end);  %year is last four digits
      | 
      | last = get_param(sys,'LastModifiedDate');
      | if isempty(last)
      |     last = datestr(now,'yyyy');
      | else
      |     last = last(end-3:end);
      | end
      | 
      | if strcmp(first,last)
      |     fprintf('%s -- Copyright %s Nexteer',NxtrConf,first)
      | else
      |     fprintf('%s -- %s%s- %s Nexteer',NxtrConf,char(169),first,last)
      | end
  Spi_WriteIB : Subsystem
  wires:
  Constant2/1 -> Call_Spi_AsyncTransmit/1(Sequence)
  Constant5/1 -> Spi_WriteIB/2(DataBufferPtr)
  Constant3/1 -> Spi_WriteIB/1(Channel)

== system ES008A_PwrSply/PwrSply/PwrSplyPer1/SysSt = Enable/PwrSplyReadWrOrderFlg1 = 0 (Write Cmd to get Diag Status) /Read Message 2 ==
  note: 4096
  note: Read Cmd: Diag Reg 1: 00100 0 0 00000000
  note: Channel 1 --> for Write Cmd
      | Channel 2 --> for Diag Register 0
      | Channel 3 --> for Diag Register 1
  Call_Spi_AsyncTransmit : Subsystem
  Constant10 : Constant  Value=PWRSPLYDIAGREG1READVAL_CNT_U16
  Constant8 : Constant  Value=SpiConf_SpiSequence_PwrSplySeq3
  Constant9 : Constant  Value=SpiConf_SpiChannel_PwrSplyCh3
  CopyRight1 : Subsystem  Description=|  mask(Copyright Information){none=on}
      | Copyright info block.                                               
      |                                                                     
      | Place copyright information at the top of every subsystem in design.
      mask prompts: none "No parameters"
      mask help: Place copyright information at the top of every subsystem in design.
      mask Display:
      | NxtrConf = 'Nexteer Confidential';
      | 
      | sys = bdroot; %handle for the current model ("system")
      | first = get_param(sys,'Created');
      | first = first(end-3:end);  %year is last four digits
      | 
      | last = get_param(sys,'LastModifiedDate');
      | if isempty(last)
      |     last = datestr(now,'yyyy');
      | else
      |     last = last(end-3:end);
      | end
      | 
      | if strcmp(first,last)
      |     fprintf('%s -- Copyright %s Nexteer',NxtrConf,first)
      | else
      |     fprintf('%s -- %s%s- %s Nexteer',NxtrConf,char(169),first,last)
      | end
  Spi_WriteIB : Subsystem
  wires:
  Constant8/1 -> Call_Spi_AsyncTransmit/1(Sequence)
  Constant10/1 -> Spi_WriteIB/2(DataBufferPtr)
  Constant9/1 -> Spi_WriteIB/1(Channel)

== system ES008A_PwrSply/PwrSply/PwrSplyPer1/SysSt = Enable/PwrSplyReadWrOrderFlg1 = 0 (Write Cmd to get Diag Status) /Write Message 1 ==
  note: (Dummy) Write Cmd: 00110 1 0 00000000
  Call_Spi_AsyncTransmit : Subsystem
  Constant4 : Constant  Value=SpiConf_SpiSequence_PwrSplySeq1
  Constant6 : Constant  Value=SpiConf_SpiChannel_PwrSplyCh1
  Constant7 : Constant  Value=PWRSPLYOUTPENAWRVAL_CNT_U16
  CopyRight1 : Subsystem  Description=|  mask(Copyright Information){none=on}
      | Copyright info block.                                               
      |                                                                     
      | Place copyright information at the top of every subsystem in design.
      mask prompts: none "No parameters"
      mask help: Place copyright information at the top of every subsystem in design.
      mask Display:
      | NxtrConf = 'Nexteer Confidential';
      | 
      | sys = bdroot; %handle for the current model ("system")
      | first = get_param(sys,'Created');
      | first = first(end-3:end);  %year is last four digits
      | 
      | last = get_param(sys,'LastModifiedDate');
      | if isempty(last)
      |     last = datestr(now,'yyyy');
      | else
      |     last = last(end-3:end);
      | end
      | 
      | if strcmp(first,last)
      |     fprintf('%s -- Copyright %s Nexteer',NxtrConf,first)
      | else
      |     fprintf('%s -- %s%s- %s Nexteer',NxtrConf,char(169),first,last)
      | end
  Spi_WriteIB : Subsystem
  wires:
  Constant4/1 -> Call_Spi_AsyncTransmit/1(Sequence)
  Constant7/1 -> Spi_WriteIB/2(DataBufferPtr)
  Constant6/1 -> Spi_WriteIB/1(Channel)
